simulink model "example"  (Simulink 7.7)
settings: Solver=ode45  StartTime=0.0  StopTime=10.0  RelTol=1e-3
libraries: simeventsattributes2 x4, simeventssink1 x1, simeventsgenerators1 x1, simeventsserver1 x1
settings Model: Creator=ACME  LastModifiedBy=ACME
settings SimEventsCC: propDiagAttribOutput=1  propDiagFcnCallOutput=1  propDiagStatOutput=0

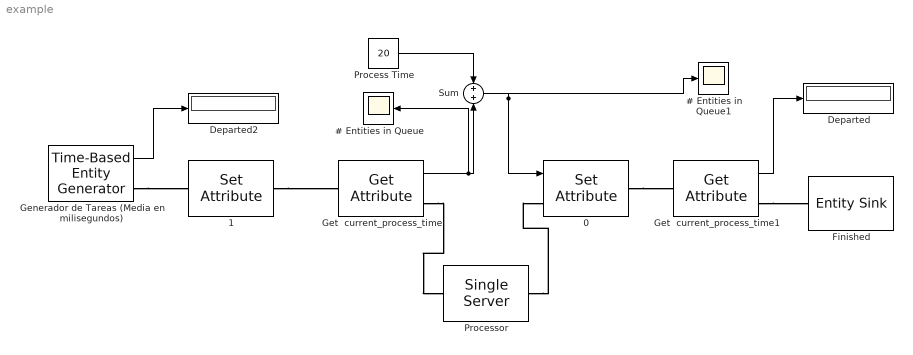
== system example ==
  # Entities in Queue : Scope
  # Entities in Queue1 : Scope
  0 : simeventsattributes2/Set Attribute  SystemSampleTime=-1  AttributeFrom=Signal port  AttributeName=A  AttributeTreatAsVector=1  AttributeValue=1  AttributeCreate=on  StatNumberDeparted=Off  EvaluatedAttributeValue={[]}
  1 : simeventsattributes2/Set Attribute  SystemSampleTime=-1  AttributeFrom=Dialog  AttributeName=A  AttributeTreatAsVector=1  AttributeValue=1  AttributeCreate=on  StatNumberDeparted=Off  EvaluatedAttributeValue={1}
  Departed : Display
  Departed2 : Display
  Finished : simeventssink1/Entity Sink  SystemSampleTime=-1  AvailableForArrivals=on  StatNumberArrived=On
  Generador de Tareas (Media en milisegundos) : simeventsgenerators1/Entity Generators/Time-Based Entity Generator  SystemSampleTime=-1  GenerateEntitiesUpon=Intergeneration time from dialog  Distribution=Constant  Minimum=0  Maximum=1  Mean=212.8  InitialSeed=1234  Period=1000000000000  PriorityEntityGeneration=300  GenerateEntityAtSimulationStart=on  ResponseWhenBlocked=Pause generation  ResponseWhenUnblocked=Immediate restart  EntityType=Blank  StatNumberDeparted=On  StatPendingEntity=Off  StatAverageIntergenerationTime=Off
  Get  current_process_time : simeventsattributes2/Get Attribute  SystemSampleTime=-1  AttributeName=A  AttributeMissing=Error  AttributeDefaultValue=1  AttributeSendTiming=After entity departure  AttributeTreatAsVector=1  StatNumberDeparted=Off  EvaluatedDefaultAttributeValue={[]}
  Get  current_process_time1 : simeventsattributes2/Get Attribute  SystemSampleTime=-1  AttributeName=A  AttributeMissing=Error  AttributeDefaultValue=1  AttributeSendTiming=After entity departure  AttributeTreatAsVector=1  StatNumberDeparted=Off  EvaluatedDefaultAttributeValue={[]}
  Process Time : Constant  Value=20
  Processor : simeventsserver1/Single Server  SystemSampleTime=-1  ServiceTimeFrom=Dialog  ServiceTime=1  AttributeName=ServiceTime  PriorityServiceCompletion=500  PermitPreemption=off  SortingAttributeName=PriorityAttributeName  SortingDirection=Ascending  WriteToAttribute=off  ResidualAttributeName=ResidualServiceTime  CreateAttribute=on  EnableTOPort=off  StatNumberDeparted=Off  StatNumberInBlock=Off  StatNumberPreempted=Off  StatPendingEntity=Off  StatAverageWait=Off  StatUtilization=Off  StatNumberTimedout=Off
  Sum : Sum
  wires:
  Process Time/1 -> Sum/1
  Get  current_process_time/1 -> Sum/2, # Entities in Queue/1
  Sum/1 -> 0/1, # Entities in Queue1/1
  Get  current_process_time1/1 -> Departed/1
  Generador de Tareas (Media en milisegundos)/1 -> Departed2/1
  connections:
  1/RConn1 -- Get  current_process_time/LConn1
  Generador de Tareas (Media en milisegundos)/RConn1 -- 1/LConn1
  Get  current_process_time1/RConn1 -- Finished/LConn1
  0/RConn1 -- Get  current_process_time1/LConn1
  Get  current_process_time/RConn1 -- Processor/LConn1
  Processor/RConn1 -- 0/LConn1
